simulink model "Optimization_Designer"  (R2022a)
settings: Solver=VariableStepAuto  StartTime=0.0  StopTime=31  MaxStep=0.01  RelTol=1e-3
undefined symbols (not defined in the file): abs_max_torque, ABS_MAX_TORQUE, ABS_MIN_TORQUE, dTx, MAX_DRIVER_INPUT, motor_enable, mu_factor, optimization_offset, Torque_Down_Rate_Limit, Torque_Up_Rate_Limit, yaw_error_limit
settings Model: FPTShortcutValueString='{{},{''BaselineRun_4'',1,1,1,''BaselineRun_4'','''',{},''M'',''D'',''''}}'  Creator=Inver  LastModifiedBy=Inver
settings DebuggingCC: SignalRangeChecking=warning

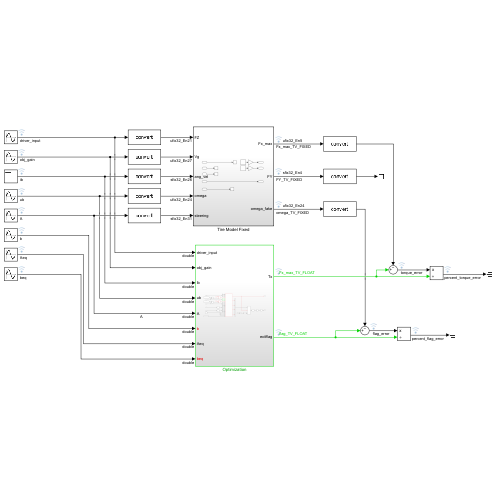
[thumbnail: Simulink's stored preview of the top-level diagram]
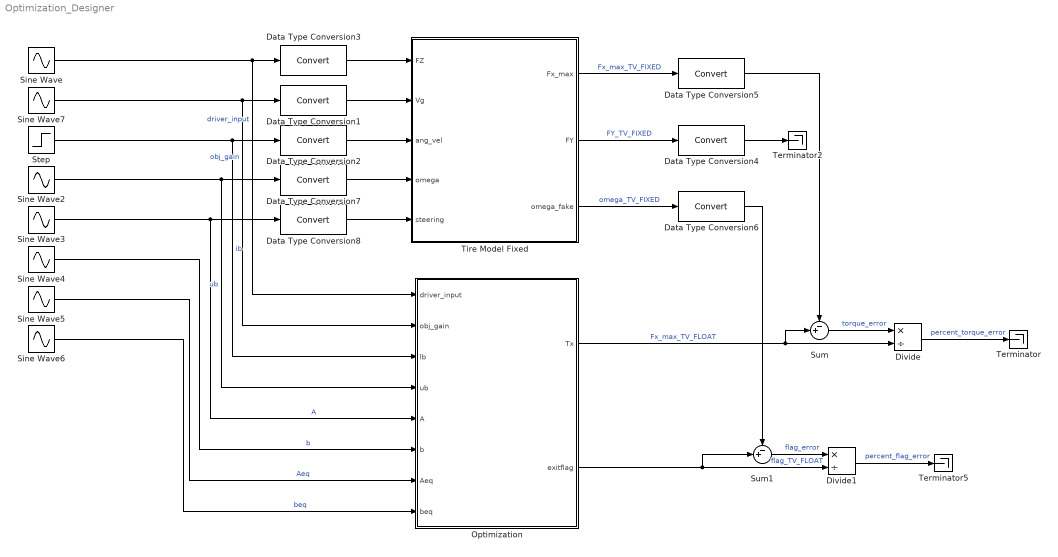
== system Optimization_Designer ==
  Data Type Conversion{1..8} (8 alike) : DataTypeConversion  SaturateOnIntegerOverflow=off  RndMeth=Floor
  Divide : Product  Inputs=*/
  Divide1 : Product  Inputs=*/
  Optimization : Subsystem
  Sine Wave : Sin  Amplitude=MAX_DRIVER_INPUT  Frequency=2*pi  SampleTime=0
  Sine Wave2 : Sin  Amplitude=ABS_MAX_TORQUE/2  Bias=ABS_MAX_TORQUE/2  Frequency=2*pi  SampleTime=0
  Sine Wave{3..7} (5 alike) : Sin  Amplitude=96  Bias=104  Frequency=2*pi  SampleTime=0
  Step : Step  After=ABS_MIN_TORQUE  SampleTime=0
  Sum : Sum  Inputs=-+|
  Sum1 : Sum  Inputs=-+|
  Terminator : Terminator
  Terminator2 : Terminator
  Terminator5 : Terminator
  Tire Model Fixed : Subsystem
  wires:
  Tire Model Fixed/2(FY) -> Data Type Conversion4/1  "FY_TV_FIXED"
  Step/1 -> Optimization/3(lb), Data Type Conversion2/1  "ib"
  Sine Wave7/1 -> Optimization/2(obj_gain), Data Type Conversion1/1  "obj_gain"
  Sine Wave/1 -> Optimization/1(driver_input), Data Type Conversion3/1  "driver_input"
  Data Type Conversion1/1 -> Tire Model Fixed/2(Vg)
  Optimization/1(Tx) -> Sum/2, Divide/2  "Fx_max_TV_FLOAT"
  Data Type Conversion3/1 -> Tire Model Fixed/1(FZ)
  Data Type Conversion2/1 -> Tire Model Fixed/3(ang_vel)
  Data Type Conversion5/1 -> Sum/1
  Sum/1 -> Divide/1  "torque_error"
  Divide/1 -> Terminator/1  "percent_torque_error"
  Tire Model Fixed/1(Fx_max) -> Data Type Conversion5/1  "Fx_max_TV_FIXED"
  Tire Model Fixed/3(omega_fake) -> Data Type Conversion6/1  "omega_TV_FIXED"
  Data Type Conversion6/1 -> Sum1/1
  Data Type Conversion4/1 -> Terminator2/1
  Data Type Conversion8/1 -> Tire Model Fixed/5(steering)
  Data Type Conversion7/1 -> Tire Model Fixed/4(omega)
  Sine Wave3/1 -> Optimization/5(A), Data Type Conversion8/1  "A"
  Sine Wave2/1 -> Optimization/4(ub), Data Type Conversion7/1  "ub"
  Optimization/2(exitflag) -> Sum1/2, Divide1/2  "flag_TV_FLOAT"
  Divide1/1 -> Terminator5/1  "percent_flag_error"
  Sum1/1 -> Divide1/1  "flag_error"
  Sine Wave4/1 -> Optimization/6(b)  "b"
  Sine Wave5/1 -> Optimization/7(Aeq)  "Aeq"
  Sine Wave6/1 -> Optimization/8(beq)  "beq"

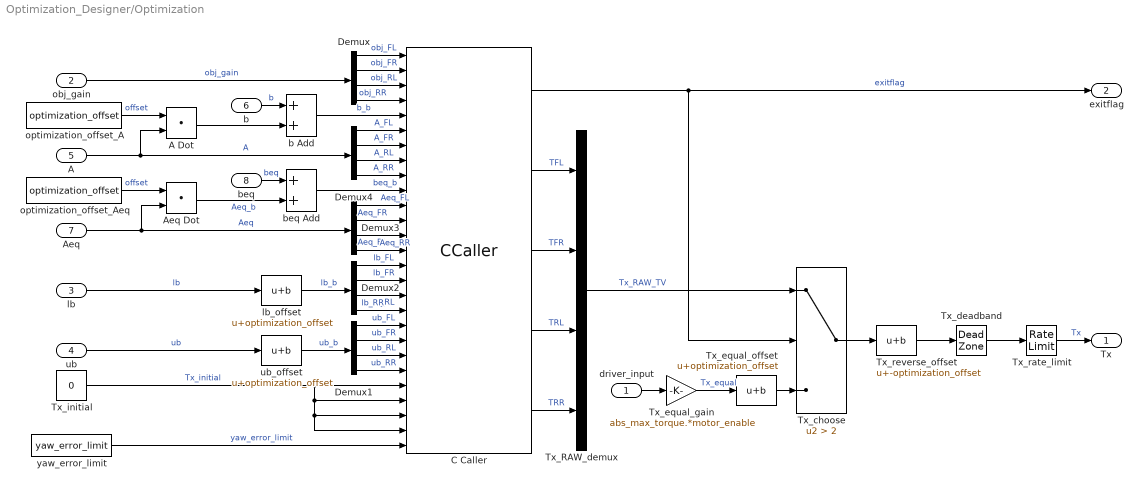
== system Optimization_Designer/Optimization ==
  driver_input : Inport  OutDataTypeStr=double
  obj_gain : Inport  Port=2
  lb : Inport  Port=3  OutDataTypeStr=double
  ub : Inport  Port=4  OutDataTypeStr=double
  A : Inport  Port=5  OutDataTypeStr=double
  b : Inport  Port=6  OutDataTypeStr=double
  Aeq : Inport  Port=7  OutDataTypeStr=double
  beq : Inport  Port=8  OutDataTypeStr=double
  A Dot : DotProduct  OutDataTypeStr=double
  Aeq Dot : DotProduct  OutDataTypeStr=double
  C Caller : CCaller  FunctionName=bigM_func  PortSpecificationStruct="%)30     .    N\"X   8    (     @         %    \"    !P    !     0         %  0 \"0    $    _    07)G3F%M90  4&]R=$YA;64 4V-O<&4     26YD97@     5'EP90      4VEZ90      27-';&]B86P   X    P    !@    @    $          4    (     0    ,    !         !   P!O=70 #@   #     &    \"     0         !0    @    !     P    $         $  # &]U=  .    .     8    (    !          %    \"     $    &     0         0  ...(+15750 chars)"
  Demux{,1..4} (5 alike) : Demux
  Tx_RAW_demux : Mux
  Tx_choose : Switch  Criteria=u2 > Threshold  Threshold=2  OutDataTypeStr=double  SaturateOnIntegerOverflow=off  InputSameDT=off
  Tx_deadband : DeadZone  LowerValue=-2*dTx  UpperValue=2*dTx  SaturateOnIntegerOverflow=off
  Tx_equal_gain : Gain  Gain=abs_max_torque.*motor_enable  OutDataTypeStr=double
  Tx_equal_offset : Bias  Bias=optimization_offset  SaturateOnIntegerOverflow=off
  Tx_initial : Constant  Value=0  OutDataTypeStr=double
  Tx_rate_limit : RateLimiter  RisingSlewLimit=Torque_Up_Rate_Limit  FallingSlewLimit=-Torque_Down_Rate_Limit  SampleTimeMode=inherited
  Tx_reverse_offset : Bias  Bias=-optimization_offset  SaturateOnIntegerOverflow=off
  b Add : Sum  OutDataTypeStr=double
  beq Add : Sum  OutDataTypeStr=double
  lb_offset : Bias  Bias=optimization_offset  SaturateOnIntegerOverflow=off
  optimization_offset_A : Constant  Value=optimization_offset  OutDataTypeStr=double
  optimization_offset_Aeq : Constant  Value=optimization_offset  OutDataTypeStr=double
  ub_offset : Bias  Bias=optimization_offset  SaturateOnIntegerOverflow=off
  yaw_error_limit : Constant  Value=yaw_error_limit  OutDataTypeStr=double
  Tx : Outport
  exitflag : Outport  Port=2
  wires:
  C Caller/1 -> Tx_choose/2, exitflag/1  "exitflag"
  lb/1 -> lb_offset/1  "lb"
  ub/1 -> ub_offset/1  "ub"
  C Caller/2 -> Tx_RAW_demux/1  "TFL"
  C Caller/5 -> Tx_RAW_demux/4  "TRR"
  C Caller/4 -> Tx_RAW_demux/3  "TRL"
  C Caller/3 -> Tx_RAW_demux/2  "TFR"
  Demux/1 -> C Caller/1  "obj_FL"
  Demux/2 -> C Caller/2  "obj_FR"
  Demux/3 -> C Caller/3  "obj_RL"
  Demux/4 -> C Caller/4  "obj_RR"
  Tx_initial/1 -> C Caller/25, C Caller/26, C Caller/24, C Caller/23  "Tx_initial"
  Demux1/1 -> C Caller/19  "ub_FL"
  Demux1/2 -> C Caller/20  "ub_FR"
  Demux1/3 -> C Caller/21  "ub_RL"
  Demux1/4 -> C Caller/22  "ub_RR"
  Demux2/1 -> C Caller/15  "lb_FL"
  Demux2/2 -> C Caller/16  "lb_FR"
  Demux2/3 -> C Caller/17  "lb_RL"
  Demux2/4 -> C Caller/18  "lb_RR"
  Demux3/3 -> C Caller/13  "Aeq_RL"
  Demux3/2 -> C Caller/12  "Aeq_FR"
  Demux3/1 -> C Caller/11  "Aeq_FL"
  Demux3/4 -> C Caller/14  "Aeq_RR"
  Demux4/1 -> C Caller/6  "A_FL"
  Demux4/2 -> C Caller/7  "A_FR"
  Demux4/3 -> C Caller/8  "A_RL"
  Demux4/4 -> C Caller/9  "A_RR"
  ub_offset/1 -> Demux1/1  "ub_b"
  optimization_offset_Aeq/1 -> Aeq Dot/1  "offset"
  optimization_offset_A/1 -> A Dot/1  "offset"
  beq/1 -> beq Add/1  "beq"
  Aeq Dot/1 -> beq Add/2  "Aeq_b"
  b/1 -> b Add/1  "b"
  A Dot/1 -> b Add/2
  yaw_error_limit/1 -> C Caller/27  "yaw_error_limit"
  Tx_RAW_demux/1 -> Tx_choose/1  "Tx_RAW_TV"
  A/1 -> Demux4/1, A Dot/2  "A"
  b Add/1 -> C Caller/5  "b_b"
  obj_gain/1 -> Demux/1  "obj_gain"
  lb_offset/1 -> Demux2/1  "lb_b"
  Aeq/1 -> Demux3/1, Aeq Dot/2  "Aeq"
  beq Add/1 -> C Caller/10  "beq_b"
  Tx_rate_limit/1 -> Tx/1  "Tx"
  Tx_reverse_offset/1 -> Tx_deadband/1
  driver_input/1 -> Tx_equal_gain/1
  Tx_deadband/1 -> Tx_rate_limit/1
  Tx_choose/1 -> Tx_reverse_offset/1
  Tx_equal_gain/1 -> Tx_equal_offset/1  "Tx_equal"
  Tx_equal_offset/1 -> Tx_choose/3

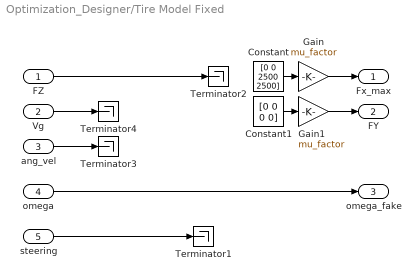
== system Optimization_Designer/Tire Model Fixed ==
  FZ : Inport  OutDataTypeStr=fixdt(0,32,21)  LockScale=on
  Vg : Inport  Port=2  OutDataTypeStr=fixdt(0,32,27)  LockScale=on
  ang_vel : Inport  Port=3  OutDataTypeStr=fixdt(1,32,26)  LockScale=on
  omega : Inport  Port=4  OutDataTypeStr=fixdt(0,32,24)  LockScale=on
  steering : Inport  Port=5  OutDataTypeStr=fixdt(1,32,31)  LockScale=on
  Constant : Constant  Value=[0 0 2500 2500]  OutDataTypeStr=fixdt(0,32,5)
  Constant1 : Constant  Value=[0 0 0 0]  OutDataTypeStr=fixdt(1,32,4)
  Gain : Gain  Gain=mu_factor  OutDataTypeStr=fixdt(0,32,5)
  Gain1 : Gain  Gain=mu_factor  OutDataTypeStr=fixdt(1,32,4)
  Terminator{1..4} (4 alike) : Terminator
  Fx_max : Outport  OutDataTypeStr=fixdt(0,32,5)  LockScale=on
  FY : Outport  Port=2  OutDataTypeStr=fixdt(1,32,4)  LockScale=on
  omega_fake : Outport  Port=3  OutDataTypeStr=fixdt(0,32,24)  LockScale=on
  wires:
  omega/1 -> omega_fake/1
  FZ/1 -> Terminator2/1
  Gain/1 -> Fx_max/1
  Gain1/1 -> FY/1
  Constant/1 -> Gain/1
  Constant1/1 -> Gain1/1
  steering/1 -> Terminator1/1
  ang_vel/1 -> Terminator3/1
  Vg/1 -> Terminator4/1
